simulink model "test_mdl_NI"  (R2018a)
settings: Solver=VariableStepAuto  StartTime=0.0  StopTime=10.0  RelTol=1e-3
(part 22 of 24)

== system test_mdl_NI/CAN_Signal/GWM/Other_GWMTx/APIM_Request_Signals_FD1/CbnCmrtPrefListIndx_Rq ==
  in : Inport
  out : Outport
  wires:
  in/1 -> out/1

== system test_mdl_NI/CAN_Signal/GWM/Other_GWMTx/APIM_Request_Signals_FD1/CbnCmrtPrefLstNmItm_Rq ==
  in : Inport
  out : Outport
  wires:
  in/1 -> out/1

== system test_mdl_NI/CAN_Signal/GWM/Other_GWMTx/APIM_Request_Signals_FD1/ChargePortPwr_Rq ==
  in : Inport
  out : Outport
  wires:
  in/1 -> out/1

== system test_mdl_NI/CAN_Signal/GWM/Other_GWMTx/APIM_Request_Signals_FD1/ChrgStatDsply_D_Rq ==
  in : Inport
  out : Outport
  wires:
  in/1 -> out/1

== system test_mdl_NI/CAN_Signal/GWM/Other_GWMTx/APIM_Request_Signals_FD1/FactoryReset_Rq ==
  in : Inport
  out : Outport
  wires:
  in/1 -> out/1

== system test_mdl_NI/CAN_Signal/GWM/Other_GWMTx/APIM_Request_Signals_FD1/LongTermParking_Rq ==
  in : Inport
  out : Outport
  wires:
  in/1 -> out/1

== system test_mdl_NI/CAN_Signal/GWM/Other_GWMTx/APIM_Request_Signals_FD1/ModemReset_D_Rq ==
  in : Inport
  out : Outport
  wires:
  in/1 -> out/1

== system test_mdl_NI/CAN_Signal/GWM/Other_GWMTx/APIM_Request_Signals_FD1/NextUsageTimeToggle_Rq ==
  in : Inport
  out : Outport
  wires:
  in/1 -> out/1

== system test_mdl_NI/CAN_Signal/GWM/Other_GWMTx/APIM_Request_Signals_FD1/OffPeakTimeSetHR_Rq ==
  in : Inport
  out : Outport
  wires:
  in/1 -> out/1

== system test_mdl_NI/CAN_Signal/GWM/Other_GWMTx/APIM_Request_Signals_FD1/OffPeakTimeSetMin_Rq ==
  in : Inport
  out : Outport
  wires:
  in/1 -> out/1

== system test_mdl_NI/CAN_Signal/GWM/Other_GWMTx/APIM_Request_Signals_FD1/StopStrtDrvMde_B_RqBtn3 ==
  in : Inport
  out : Outport
  wires:
  in/1 -> out/1

== system test_mdl_NI/CAN_Signal/GWM/Other_GWMTx/APIM_Request_Signals_FD1/TCU_ESN_D_Rq ==
  in : Inport
  out : Outport
  wires:
  in/1 -> out/1

== system test_mdl_NI/CAN_Signal/GWM/Other_GWMTx/APIM_Send_Signals1_FD1/APIM_ActiveTrackNum_St ==
  in : Inport
  out : Outport
  wires:
  in/1 -> out/1

== system test_mdl_NI/CAN_Signal/GWM/Other_GWMTx/APIM_Send_Signals1_FD1/APIM_NumberofTracks_St ==
  in : Inport
  out : Outport
  wires:
  in/1 -> out/1

== system test_mdl_NI/CAN_Signal/GWM/Other_GWMTx/APIM_Send_Signals1_FD1/AutoHoldSwtch_D_Stat3 ==
  in : Inport
  out : Outport
  wires:
  in/1 -> out/1

== system test_mdl_NI/CAN_Signal/GWM/Other_GWMTx/APIM_Send_Signals1_FD1/CenterStackRing_D_Actl ==
  in : Inport
  out : Outport
  wires:
  in/1 -> out/1

== system test_mdl_NI/CAN_Signal/GWM/Other_GWMTx/APIM_Send_Signals1_FD1/ChrgCordUnlock_B_Rq ==
  in : Inport
  out : Outport
  wires:
  in/1 -> out/1

== system test_mdl_NI/CAN_Signal/GWM/Other_GWMTx/APIM_Send_Signals1_FD1/TrlrAidCancl_B_Rq ==
  in : Inport
  out : Outport
  wires:
  in/1 -> out/1

== system test_mdl_NI/CAN_Signal/GWM/Other_GWMTx/APIM_Send_Signals1_FD1/TrlrAidSetup_D_Stat ==
  in : Inport
  out : Outport
  wires:
  in/1 -> out/1

== system test_mdl_NI/CAN_Signal/GWM/Other_GWMTx/APIM_Send_Signals1_FD1/TrlrTrgtAcquire_D_Rq ==
  in : Inport
  out : Outport
  wires:
  in/1 -> out/1

== system test_mdl_NI/CAN_Signal/GWM/Other_GWMTx/APIM_Send_Signals1_FD1/ValetMode_D_Stat ==
  in : Inport
  out : Outport
  wires:
  in/1 -> out/1

== system test_mdl_NI/CAN_Signal/GWM/Other_GWMTx/APIM_Send_Signals_2_FD1/OnbChrgClearAll_B_Rq ==
  in : Inport
  out : Outport
  wires:
  in/1 -> out/1

== system test_mdl_NI/CAN_Signal/GWM/Other_GWMTx/APIM_Send_Signals_2_FD1/OnbChrgGoTDelete_B_Rq ==
  in : Inport
  out : Outport
  wires:
  in/1 -> out/1

== system test_mdl_NI/CAN_Signal/GWM/Other_GWMTx/APIM_Send_Signals_2_FD1/OnbChrgGoTElement_D_Rq ==
  in : Inport
  out : Outport
  wires:
  in/1 -> out/1

== system test_mdl_NI/CAN_Signal/GWM/Other_GWMTx/APIM_Send_Signals_2_FD1/OnbChrgGoTExtHtr_D_Rq ==
  in : Inport
  out : Outport
  wires:
  in/1 -> out/1

== system test_mdl_NI/CAN_Signal/GWM/Other_GWMTx/APIM_Send_Signals_2_FD1/OnbChrgGoTHr_T_Rq ==
  in : Inport
  out : Outport
  wires:
  in/1 -> out/1

== system test_mdl_NI/CAN_Signal/GWM/Other_GWMTx/APIM_Send_Signals_2_FD1/OnbChrgGoTMnte_D_Rq ==
  in : Inport
  out : Outport
  wires:
  in/1 -> out/1

== system test_mdl_NI/CAN_Signal/GWM/Other_GWMTx/APIM_Send_Signals_2_FD1/OnbChrgGoTOn_D_Rq ==
  in : Inport
  out : Outport
  wires:
  in/1 -> out/1

== system test_mdl_NI/CAN_Signal/GWM/Other_GWMTx/APIM_Send_Signals_2_FD1/OnbChrgGoTPrcond_D_Rq ==
  in : Inport
  out : Outport
  wires:
  in/1 -> out/1

== system test_mdl_NI/CAN_Signal/GWM/Other_GWMTx/APIM_Send_Signals_2_FD1/OnbChrgGoTTouch_D_Rq ==
  in : Inport
  out : Outport
  wires:
  in/1 -> out/1

== system test_mdl_NI/CAN_Signal/GWM/Other_GWMTx/APIM_Send_Signals_2_FD1/OnbChrgGoTUpdate_B_Rq ==
  in : Inport
  out : Outport
  wires:
  in/1 -> out/1

== system test_mdl_NI/CAN_Signal/GWM/Other_GWMTx/APIM_Send_Signals_2_FD1/OtaTrg_D_Stat ==
  in : Inport
  out : Outport
  wires:
  in/1 -> out/1

== system test_mdl_NI/CAN_Signal/GWM/Other_GWMTx/APIM_Send_Signals_2_FD1/PaakMyKey_D_Rq ==
  in : Inport
  out : Outport
  wires:
  in/1 -> out/1

== system test_mdl_NI/CAN_Signal/GWM/Other_GWMTx/APIM_Send_Signals_2_FD1/TCU_Final_Actvtn_St ==
  in : Inport
  out : Outport
  wires:
  in/1 -> out/1

== system test_mdl_NI/CAN_Signal/GWM/Other_GWMTx/APIM_Send_Signals_2_FD1/TCU_Init_Actvtn_St ==
  in : Inport
  out : Outport
  wires:
  in/1 -> out/1

== system test_mdl_NI/CAN_Signal/GWM/Other_GWMTx/APIM_Send_Signals_2_FD1/TrlrAidMde_D_Rq ==
  in : Inport
  out : Outport
  wires:
  in/1 -> out/1

== system test_mdl_NI/CAN_Signal/GWM/Other_GWMTx/ActiveFrontStrg_Stat2_FD1/SteWhlRelCalib_An_Sns ==
  in : Inport
  out : Outport
  wires:
  in/1 -> out/1

== system test_mdl_NI/CAN_Signal/GWM/Other_GWMTx/ActiveFrontStrg_Stat2_FD1/SteWhlRelCalib_T_Actl ==
  in : Inport
  out : Outport
  wires:
  in/1 -> out/1

== system test_mdl_NI/CAN_Signal/GWM/Other_GWMTx/ActiveFrontStrg_Stat_FD1/SteWhlBrkAnActl_No_Cnt ==
  in : Inport
  out : Outport
  wires:
  in/1 -> out/1

== system test_mdl_NI/CAN_Signal/GWM/Other_GWMTx/ActiveFrontStrg_Stat_FD1/SteWhlBrkAnActl_No_Cs ==
  in : Inport
  out : Outport
  wires:
  in/1 -> out/1

== system test_mdl_NI/CAN_Signal/GWM/Other_GWMTx/ActiveFrontStrg_Stat_FD1/SteWhlBrkOffst_An_Actl ==
  in : Inport
  out : Outport
  wires:
  in/1 -> out/1

== system test_mdl_NI/CAN_Signal/GWM/Other_GWMTx/ActiveFrontStrg_Stat_FD1/SteWhlOffstRq_D_Stat ==
  in : Inport
  out : Outport
  wires:
  in/1 -> out/1

== system test_mdl_NI/CAN_Signal/GWM/Other_GWMTx/ActiveFrontStrg_Stat_FD1/SteWhlOffst_An_TotActl ==
  in : Inport
  out : Outport
  wires:
  in/1 -> out/1

== system test_mdl_NI/CAN_Signal/GWM/Other_GWMTx/AllTerrainControlData_FD1/SelDrvMdeCnt_D_Stat ==
  in : Inport
  out : Outport
  wires:
  in/1 -> out/1

== system test_mdl_NI/CAN_Signal/GWM/Other_GWMTx/AllTerrainControlData_FD1/SelDrvMdeSwtchOk_D_Stat ==
  in : Inport
  out : Outport
  wires:
  in/1 -> out/1

== system test_mdl_NI/CAN_Signal/GWM/Other_GWMTx/AllTerrainControlData_FD1/SelDrvMdeSwtch_D_Stat ==
  in : Inport
  out : Outport
  wires:
  in/1 -> out/1

== system test_mdl_NI/CAN_Signal/GWM/Other_GWMTx/AllTerrainControlData_FD1/SelDrvMdeSwtch_No_Actl ==
  in : Inport
  out : Outport
  wires:
  in/1 -> out/1

== system test_mdl_NI/CAN_Signal/GWM/Other_GWMTx/All_Terrain_Data_FD1/TerrMde_D_RqDrv ==
  in : Inport
  out : Outport
  wires:
  in/1 -> out/1

== system test_mdl_NI/CAN_Signal/GWM/Other_GWMTx/All_Terrain_Data_FD1/TerrStat_D_RqDsply ==
  in : Inport
  out : Outport
  wires:
  in/1 -> out/1

== system test_mdl_NI/CAN_Signal/GWM/Other_GWMTx/BCM_Lamp_Stat_FD1/BrkWarnInd_B_Rq ==
  in : Inport
  out : Outport
  wires:
  in/1 -> out/1

== system test_mdl_NI/CAN_Signal/GWM/Other_GWMTx/BCM_Lamp_Stat_FD1/Brk_Fluid_Lvl_Low ==
  in : Inport
  out : Outport
  wires:
  in/1 -> out/1

== system test_mdl_NI/CAN_Signal/GWM/Other_GWMTx/BCM_Lamp_Stat_FD1/Courtesy_BSave_Stat ==
  in : Inport
  out : Outport
  wires:
  in/1 -> out/1

== system test_mdl_NI/CAN_Signal/GWM/Other_GWMTx/BCM_Lamp_Stat_FD1/Courtesy_Delay_Status ==
  in : Inport
  out : Outport
  wires:
  in/1 -> out/1

== system test_mdl_NI/CAN_Signal/GWM/Other_GWMTx/BCM_Lamp_Stat_FD1/CrnrLghtLeft_Pc_Rq ==
  in : Inport
  out : Outport
  wires:
  in/1 -> out/1

== system test_mdl_NI/CAN_Signal/GWM/Other_GWMTx/BCM_Lamp_Stat_FD1/CrnrLghtRight_Pc_Rq ==
  in : Inport
  out : Outport
  wires:
  in/1 -> out/1

== system test_mdl_NI/CAN_Signal/GWM/Other_GWMTx/BCM_Lamp_Stat_FD1/DayRnngLampOn_B_Stat ==
  in : Inport
  out : Outport
  wires:
  in/1 -> out/1

== system test_mdl_NI/CAN_Signal/GWM/Other_GWMTx/BCM_Lamp_Stat_FD1/DrTgateLck_D_Stat ==
  in : Inport
  out : Outport
  wires:
  in/1 -> out/1

== system test_mdl_NI/CAN_Signal/GWM/Other_GWMTx/BCM_Lamp_Stat_FD1/Dr_Courtesy_Light_Stat ==
  in : Inport
  out : Outport
  wires:
  in/1 -> out/1

== system test_mdl_NI/CAN_Signal/GWM/Other_GWMTx/BCM_Lamp_Stat_FD1/HeadLampLoActv_B_Stat ==
  in : Inport
  out : Outport
  wires:
  in/1 -> out/1

== system test_mdl_NI/CAN_Signal/GWM/Other_GWMTx/BCM_Lamp_Stat_FD1/HeadLampLoFlOn_B_Stat ==
  in : Inport
  out : Outport
  wires:
  in/1 -> out/1

== system test_mdl_NI/CAN_Signal/GWM/Other_GWMTx/BCM_Lamp_Stat_FD1/HeadLampLoFrOn_B_Stat ==
  in : Inport
  out : Outport
  wires:
  in/1 -> out/1

== system test_mdl_NI/CAN_Signal/GWM/Other_GWMTx/BCM_Lamp_Stat_FD1/HeadLampLoOut_B_Stat ==
  in : Inport
  out : Outport
  wires:
  in/1 -> out/1

== system test_mdl_NI/CAN_Signal/GWM/Other_GWMTx/BCM_Lamp_Stat_FD1/HeadLghtHiFdbck_D_Stat ==
  in : Inport
  out : Outport
  wires:
  in/1 -> out/1

== system test_mdl_NI/CAN_Signal/GWM/Other_GWMTx/BCM_Lamp_Stat_FD1/HeadLghtHiOn_B_Stat ==
  in : Inport
  out : Outport
  wires:
  in/1 -> out/1

== system test_mdl_NI/CAN_Signal/GWM/Other_GWMTx/BCM_Lamp_Stat_FD1/HeadLghtSwtch_D_Stat ==
  in : Inport
  out : Outport
  wires:
  in/1 -> out/1

== system test_mdl_NI/CAN_Signal/GWM/Other_GWMTx/BCM_Lamp_Stat_FD1/Headlamp_On_Wrning_Cmd ==
  in : Inport
  out : Outport
  wires:
  in/1 -> out/1

== system test_mdl_NI/CAN_Signal/GWM/Other_GWMTx/BCM_Lamp_Stat_FD1/HomeSafeLtChime_B_Rq ==
  in : Inport
  out : Outport
  wires:
  in/1 -> out/1

== system test_mdl_NI/CAN_Signal/GWM/Other_GWMTx/BCM_Lamp_Stat_FD1/Illuminated_Entry_Stat ==
  in : Inport
  out : Outport
  wires:
  in/1 -> out/1

== system test_mdl_NI/CAN_Signal/GWM/Other_GWMTx/BCM_Lamp_Stat_FD1/ImpactEvntFdbck_D_Stat ==
  in : Inport
  out : Outport
  wires:
  in/1 -> out/1

== system test_mdl_NI/CAN_Signal/GWM/Other_GWMTx/BCM_Lamp_Stat_FD1/KeyInIgnWarn_B_Cmd ==
  in : Inport
  out : Outport
  wires:
  in/1 -> out/1

== system test_mdl_NI/CAN_Signal/GWM/Other_GWMTx/BCM_Lamp_Stat_FD1/Park_Brake_Chime_Rqst ==
  in : Inport
  out : Outport
  wires:
  in/1 -> out/1

== system test_mdl_NI/CAN_Signal/GWM/Other_GWMTx/BCM_Lamp_Stat_FD1/PerimeterAlarmChimeRq ==
  in : Inport
  out : Outport
  wires:
  in/1 -> out/1

== system test_mdl_NI/CAN_Signal/GWM/Other_GWMTx/BCM_Lamp_Stat_FD1/Perimeter_Alarm_Status ==
  in : Inport
  out : Outport
  wires:
  in/1 -> out/1

== system test_mdl_NI/CAN_Signal/GWM/Other_GWMTx/BCM_Lamp_Stat_FD1/PrkLght_D_Stat ==
  in : Inport
  out : Outport
  wires:
  in/1 -> out/1

== system test_mdl_NI/CAN_Signal/GWM/Other_GWMTx/BCM_Lamp_Stat_FD1/PrkLightChime_B_Rq ==
  in : Inport
  out : Outport
  wires:
  in/1 -> out/1

== system test_mdl_NI/CAN_Signal/GWM/Other_GWMTx/BCM_Lamp_Stat_FD1/PudLampDrv_D_Rq ==
  in : Inport
  out : Outport
  wires:
  in/1 -> out/1

== system test_mdl_NI/CAN_Signal/GWM/Other_GWMTx/BCM_Lamp_Stat_FD1/PudLampPsngr_D_Rq ==
  in : Inport
  out : Outport
  wires:
  in/1 -> out/1

== system test_mdl_NI/CAN_Signal/GWM/Other_GWMTx/BCM_Lamp_Stat_FD1/PudLamp_D_Rq ==
  in : Inport
  out : Outport
  wires:
  in/1 -> out/1

== system test_mdl_NI/CAN_Signal/GWM/Other_GWMTx/BCM_Lamp_Stat_FD1/ReducedGuard_D_Stat ==
  in : Inport
  out : Outport
  wires:
  in/1 -> out/1

== system test_mdl_NI/CAN_Signal/GWM/Other_GWMTx/BCM_Lamp_Stat_FD1/RvrseLghtOn_B_Stat ==
  in : Inport
  out : Outport
  wires:
  in/1 -> out/1

== system test_mdl_NI/CAN_Signal/GWM/Other_GWMTx/BCM_Lamp_Stat_FD1/StopLghtOn_B_Stat ==
  in : Inport
  out : Outport
  wires:
  in/1 -> out/1

== system test_mdl_NI/CAN_Signal/GWM/Other_GWMTx/BCM_Lamp_Stat_FD1/TrnNotInPrkChime_B_Rq ==
  in : Inport
  out : Outport
  wires:
  in/1 -> out/1

== system test_mdl_NI/CAN_Signal/GWM/Other_GWMTx/BCM_Lamp_Stat_FD1/WndwGlbl_D_Cmd ==
  in : Inport
  out : Outport
  wires:
  in/1 -> out/1

== system test_mdl_NI/CAN_Signal/GWM/Other_GWMTx/BCM_Lamp_Stat_FD1/WrlssAcsyChrgInhbt_B_Rq ==
  in : Inport
  out : Outport
  wires:
  in/1 -> out/1

== system test_mdl_NI/CAN_Signal/GWM/Other_GWMTx/BatteryCharge_Data2_FD1/ChrgCrdLck_D_Falt ==
  in : Inport
  out : Outport
  wires:
  in/1 -> out/1

== system test_mdl_NI/CAN_Signal/GWM/Other_GWMTx/Battery_Mgmt_24V_FD1/BattULo24Soc_Pc_Actl ==
  in : Inport
  out : Outport
  wires:
  in/1 -> out/1

== system test_mdl_NI/CAN_Signal/GWM/Other_GWMTx/Battery_Mgmt_24V_FD1/BattULo24State_D_Qlty ==
  in : Inport
  out : Outport
  wires:
  in/1 -> out/1

== system test_mdl_NI/CAN_Signal/GWM/Other_GWMTx/Battery_Mgmt_24V_FD1/BattULo24_Ah_DeltaRide ==
  in : Inport
  out : Outport
  wires:
  in/1 -> out/1

== system test_mdl_NI/CAN_Signal/GWM/Other_GWMTx/Battery_Mgmt_24V_FD1/BattULo24_B_Falt ==
  in : Inport
  out : Outport
  wires:
  in/1 -> out/1

== system test_mdl_NI/CAN_Signal/GWM/Other_GWMTx/Battery_Mgmt_24V_FD1/BattULo24_I_Actl ==
  in : Inport
  out : Outport
  wires:
  in/1 -> out/1

== system test_mdl_NI/CAN_Signal/GWM/Other_GWMTx/Battery_Mgmt_2_FD1/BattULoChrg_D_Rq ==
  in : Inport
  out : Outport
  wires:
  in/1 -> out/1

== system test_mdl_NI/CAN_Signal/GWM/Other_GWMTx/Battery_Mgmt_2_FD1/BattULoSrvc_T_Actl ==
  in : Inport
  out : Outport
  wires:
  in/1 -> out/1

== system test_mdl_NI/CAN_Signal/GWM/Other_GWMTx/Battery_Mgmt_2_FD1/Batt_Crit_SoC_B ==
  in : Inport
  out : Outport
  wires:
  in/1 -> out/1

== system test_mdl_NI/CAN_Signal/GWM/Other_GWMTx/Battery_Mgmt_2_FD1/Batt_Lo_SoC_B ==
  in : Inport
  out : Outport
  wires:
  in/1 -> out/1

== system test_mdl_NI/CAN_Signal/GWM/Other_GWMTx/Battery_Mgmt_2_FD1/ChargeMode ==
  in : Inport
  out : Outport
  wires:
  in/1 -> out/1

== system test_mdl_NI/CAN_Signal/GWM/Other_GWMTx/Battery_Mgmt_2_FD1/EngStrtInhbt_B_RqBatt ==
  in : Inport
  out : Outport
  wires:
  in/1 -> out/1

== system test_mdl_NI/CAN_Signal/GWM/Other_GWMTx/Battery_Mgmt_2_FD1/IdleSpeedIncrease_El ==
  in : Inport
  out : Outport
  wires:
  in/1 -> out/1

== system test_mdl_NI/CAN_Signal/GWM/Other_GWMTx/Battery_Mgmt_2_FD1/PeriodicElLoad_B_Stat ==
  in : Inport
  out : Outport
  wires:
  in/1 -> out/1

== system test_mdl_NI/CAN_Signal/GWM/Other_GWMTx/Battery_Mgmt_2_FD1/PwSysULoFalt_D_Stat ==
  in : Inport
  out : Outport
  wires:
  in/1 -> out/1

== system test_mdl_NI/CAN_Signal/GWM/Other_GWMTx/Battery_Mgmt_2_FD1/Shed_Drain_Eng_Off_B ==
  in : Inport
  out : Outport
  wires:
  in/1 -> out/1

== system test_mdl_NI/CAN_Signal/GWM/Other_GWMTx/Battery_Mgmt_2_FD1/Shed_Feature_Group_ID ==
  in : Inport
  out : Outport
  wires:
  in/1 -> out/1

== system test_mdl_NI/CAN_Signal/GWM/Other_GWMTx/Battery_Mgmt_2_FD1/Shed_Level_Req ==
  in : Inport
  out : Outport
  wires:
  in/1 -> out/1

== system test_mdl_NI/CAN_Signal/GWM/Other_GWMTx/Battery_Mgmt_2_FD1/Shed_T_Eng_Off_B ==
  in : Inport
  out : Outport
  wires:
  in/1 -> out/1

== system test_mdl_NI/CAN_Signal/GWM/Other_GWMTx/Battery_Mgmt_2_FD1/ULoRgenTestMde_B_Rq ==
  in : Inport
  out : Outport
  wires:
  in/1 -> out/1

== system test_mdl_NI/CAN_Signal/GWM/Other_GWMTx/Battery_Mgmt_3_FD1/BSBattQCapAh ==
  in : Inport
  out : Outport
  wires:
  in/1 -> out/1

== system test_mdl_NI/CAN_Signal/GWM/Other_GWMTx/Battery_Mgmt_3_FD1/BSBattQDeltaRideAh ==
  in : Inport
  out : Outport
  wires:
  in/1 -> out/1

== system test_mdl_NI/CAN_Signal/GWM/Other_GWMTx/Battery_Mgmt_3_FD1/BSBattSOC ==
  in : Inport
  out : Outport
  wires:
  in/1 -> out/1

== system test_mdl_NI/CAN_Signal/GWM/Other_GWMTx/Battery_Mgmt_3_FD1/BSFault ==
  in : Inport
  out : Outport
  wires:
  in/1 -> out/1

== system test_mdl_NI/CAN_Signal/GWM/Other_GWMTx/Battery_Mgmt_3_FD1/BattULo2_Te_Actl ==
  in : Inport
  out : Outport
  wires:
  in/1 -> out/1

== system test_mdl_NI/CAN_Signal/GWM/Other_GWMTx/Battery_Mgmt_3_FD1/BattULoChrg_URate_RqMx ==
  in : Inport
  out : Outport
  wires:
  in/1 -> out/1

== system test_mdl_NI/CAN_Signal/GWM/Other_GWMTx/Battery_Mgmt_3_FD1/BattULoChrg_U_RqMn ==
  in : Inport
  out : Outport
  wires:
  in/1 -> out/1

== system test_mdl_NI/CAN_Signal/GWM/Other_GWMTx/Battery_Mgmt_3_FD1/BattULoChrg_U_RqMx ==
  in : Inport
  out : Outport
  wires:
  in/1 -> out/1

== system test_mdl_NI/CAN_Signal/GWM/Other_GWMTx/Battery_Mgmt_3_FD1/BattULoState_D_Qlty ==
  in : Inport
  out : Outport
  wires:
  in/1 -> out/1

== system test_mdl_NI/CAN_Signal/GWM/Other_GWMTx/Battery_Mgmt_4_FD1/BattULoAuxSoc_Pc_Actl ==
  in : Inport
  out : Outport
  wires:
  in/1 -> out/1

== system test_mdl_NI/CAN_Signal/GWM/Other_GWMTx/Battery_Mgmt_4_FD1/BattULoAux_B_Falt ==
  in : Inport
  out : Outport
  wires:
  in/1 -> out/1

== system test_mdl_NI/CAN_Signal/GWM/Other_GWMTx/Battery_Mgmt_4_FD1/BattULoAux_D_Qlty ==
  in : Inport
  out : Outport
  wires:
  in/1 -> out/1

== system test_mdl_NI/CAN_Signal/GWM/Other_GWMTx/Battery_Mgmt_4_FD1/BattULoAux_I_Actl ==
  in : Inport
  out : Outport
  wires:
  in/1 -> out/1

== system test_mdl_NI/CAN_Signal/GWM/Other_GWMTx/Battery_Mgmt_4_FD1/BattULoAux_U_Actl ==
  in : Inport
  out : Outport
  wires:
  in/1 -> out/1

== system test_mdl_NI/CAN_Signal/GWM/Other_GWMTx/Battery_Mgmt_4_FD1/BattULoCrnkBelt_U_Pred ==
  in : Inport
  out : Outport
  wires:
  in/1 -> out/1

== system test_mdl_NI/CAN_Signal/GWM/Other_GWMTx/Battery_Mgmt_4_FD1/BattULoCrnkStrt_U_Pred ==
  in : Inport
  out : Outport
  wires:
  in/1 -> out/1

== system test_mdl_NI/CAN_Signal/GWM/Other_GWMTx/Battery_Traction_1_FD1/BattTracMil_D_Rq ==
  in : Inport
  out : Outport
  wires:
  in/1 -> out/1

== system test_mdl_NI/CAN_Signal/GWM/Other_GWMTx/Battery_Traction_1_FD1/BattTracOffFst_D_Actl ==
  in : Inport
  out : Outport
  wires:
  in/1 -> out/1

== system test_mdl_NI/CAN_Signal/GWM/Other_GWMTx/Battery_Traction_1_FD1/BattTracOff_B_Actl ==
  in : Inport
  out : Outport
  wires:
  in/1 -> out/1

== system test_mdl_NI/CAN_Signal/GWM/Other_GWMTx/Battery_Traction_1_FD1/BattTrac_I_Actl ==
  in : Inport
  out : Outport
  wires:
  in/1 -> out/1

== system test_mdl_NI/CAN_Signal/GWM/Other_GWMTx/Battery_Traction_1_FD1/BattTrac_U_Actl ==
  in : Inport
  out : Outport
  wires:
  in/1 -> out/1

== system test_mdl_NI/CAN_Signal/GWM/Other_GWMTx/Battery_Traction_1_FD1/BattTrac_U_LimHi ==
  in : Inport
  out : Outport
  wires:
  in/1 -> out/1

== system test_mdl_NI/CAN_Signal/GWM/Other_GWMTx/Battery_Traction_1_FD1/BattTrac_U_LimLo ==
  in : Inport
  out : Outport
  wires:
  in/1 -> out/1

== system test_mdl_NI/CAN_Signal/GWM/Other_GWMTx/Battery_Traction_1_FD1/VehStrtInhbt_B_RqBatt ==
  in : Inport
  out : Outport
  wires:
  in/1 -> out/1

== system test_mdl_NI/CAN_Signal/GWM/Other_GWMTx/Battery_Traction_3_FD1/BattTracClnt_Te_Actl ==
  in : Inport
  out : Outport
  wires:
  in/1 -> out/1

== system test_mdl_NI/CAN_Signal/GWM/Other_GWMTx/Battery_Traction_3_FD1/BattTracSoc_Pc_LimHi ==
  in : Inport
  out : Outport
  wires:
  in/1 -> out/1

== system test_mdl_NI/CAN_Signal/GWM/Other_GWMTx/Battery_Traction_3_FD1/BattTracSoc_Pc_LimLo ==
  in : Inport
  out : Outport
  wires:
  in/1 -> out/1

== system test_mdl_NI/CAN_Signal/GWM/Other_GWMTx/Battery_Traction_3_FD1/BattTracSoc_Pc_MnPrtct ==
  in : Inport
  out : Outport
  wires:
  in/1 -> out/1

== system test_mdl_NI/CAN_Signal/GWM/Other_GWMTx/Battery_Traction_3_FD1/BattTracSoc_Pc_MxPrtct ==
  in : Inport
  out : Outport
  wires:
  in/1 -> out/1

== system test_mdl_NI/CAN_Signal/GWM/Other_GWMTx/Battery_Traction_3_FD1/BattTracSrvcRqd_B_Rq ==
  in : Inport
  out : Outport
  wires:
  in/1 -> out/1

== system test_mdl_NI/CAN_Signal/GWM/Other_GWMTx/Battery_Traction_3_FD1/BattTracWarnLamp_B_Rq ==
  in : Inport
  out : Outport
  wires:
  in/1 -> out/1

== system test_mdl_NI/CAN_Signal/GWM/Other_GWMTx/Battery_Traction_4_FD1/BattTracDiagClr_B_Rq ==
  in : Inport
  out : Outport
  wires:
  in/1 -> out/1

== system test_mdl_NI/CAN_Signal/GWM/Other_GWMTx/Battery_Traction_4_FD1/BattTracSoc2_Pc_Actl ==
  in : Inport
  out : Outport
  wires:
  in/1 -> out/1

== system test_mdl_NI/CAN_Signal/GWM/Other_GWMTx/Battery_Traction_4_FD1/BattTrac_Te_Actl ==
  in : Inport
  out : Outport
  wires:
  in/1 -> out/1

== system test_mdl_NI/CAN_Signal/GWM/Other_GWMTx/Battery_Traction_5_FD1/BattTrac2_Pw_ChrgInst ==
  in : Inport
  out : Outport
  wires:
  in/1 -> out/1

== system test_mdl_NI/CAN_Signal/GWM/Other_GWMTx/Battery_Traction_5_FD1/BattTrac2_Pw_DchrgInst ==
  in : Inport
  out : Outport
  wires:
  in/1 -> out/1

== system test_mdl_NI/CAN_Signal/GWM/Other_GWMTx/Battery_Traction_5_FD1/BattTrac2_Pw_LimChrg ==
  in : Inport
  out : Outport
  wires:
  in/1 -> out/1

== system test_mdl_NI/CAN_Signal/GWM/Other_GWMTx/Battery_Traction_5_FD1/BattTrac2_Pw_LimDchrg ==
  in : Inport
  out : Outport
  wires:
  in/1 -> out/1

== system test_mdl_NI/CAN_Signal/GWM/Other_GWMTx/Battery_Traction_6_FD1/BattTracClntPmp_D_Stat ==
  in : Inport
  out : Outport
  wires:
  in/1 -> out/1

== system test_mdl_NI/CAN_Signal/GWM/Other_GWMTx/Battery_Traction_6_FD1/BattTracCnnct_D_Cmd ==
  in : Inport
  out : Outport
  wires:
  in/1 -> out/1

== system test_mdl_NI/CAN_Signal/GWM/Other_GWMTx/Battery_Traction_6_FD1/BattTracDcdcDis_B_Rq ==
  in : Inport
  out : Outport
  wires:
  in/1 -> out/1

== system test_mdl_NI/CAN_Signal/GWM/Other_GWMTx/Battery_Traction_6_FD1/BattTracDelta_Te_Actl ==
  in : Inport
  out : Outport
  wires:
  in/1 -> out/1

== system test_mdl_NI/CAN_Signal/GWM/Other_GWMTx/Battery_Traction_6_FD1/BattTracHvilOpen_B_Stat ==
  in : Inport
  out : Outport
  wires:
  in/1 -> out/1

== system test_mdl_NI/CAN_Signal/GWM/Other_GWMTx/Battery_Traction_6_FD1/HtrnClntPump_D_Stat ==
  in : Inport
  out : Outport
  wires:
  in/1 -> out/1

== system test_mdl_NI/CAN_Signal/GWM/Other_GWMTx/BodyInfo_3_FD1/Backlit_LED_Status ==
  in : Inport
  out : Outport
  wires:
  in/1 -> out/1

== system test_mdl_NI/CAN_Signal/GWM/Other_GWMTx/BodyInfo_3_FD1/BodySrvcRqd_B_Rq ==
  in : Inport
  out : Outport
  wires:
  in/1 -> out/1

== system test_mdl_NI/CAN_Signal/GWM/Other_GWMTx/BodyInfo_3_FD1/CrashEvnt_D_Stat ==
  in : Inport
  out : Outport
  wires:
  in/1 -> out/1

== system test_mdl_NI/CAN_Signal/GWM/Other_GWMTx/BodyInfo_3_FD1/Day_Night_Status ==
  in : Inport
  out : Outport
  wires:
  in/1 -> out/1

== system test_mdl_NI/CAN_Signal/GWM/Other_GWMTx/BodyInfo_3_FD1/Delay_Accy ==
  in : Inport
  out : Outport
  wires:
  in/1 -> out/1

== system test_mdl_NI/CAN_Signal/GWM/Other_GWMTx/BodyInfo_3_FD1/DimmingLvlEvnt_No_Actl ==
  in : Inport
  out : Outport
  wires:
  in/1 -> out/1

== system test_mdl_NI/CAN_Signal/GWM/Other_GWMTx/BodyInfo_3_FD1/Dimming_Lvl ==
  in : Inport
  out : Outport
  wires:
  in/1 -> out/1

== system test_mdl_NI/CAN_Signal/GWM/Other_GWMTx/BodyInfo_3_FD1/DrStatDrvErrCnt_B_Stat ==
  in : Inport
  out : Outport
  wires:
  in/1 -> out/1

== system test_mdl_NI/CAN_Signal/GWM/Other_GWMTx/BodyInfo_3_FD1/DrStatDrv_B_Actl ==
  in : Inport
  out : Outport
  wires:
  in/1 -> out/1

== system test_mdl_NI/CAN_Signal/GWM/Other_GWMTx/BodyInfo_3_FD1/DrStatHood_B_Actl ==
  in : Inport
  out : Outport
  wires:
  in/1 -> out/1

== system test_mdl_NI/CAN_Signal/GWM/Other_GWMTx/BodyInfo_3_FD1/DrStatInnrTgate_B_Actl ==
  in : Inport
  out : Outport
  wires:
  in/1 -> out/1

== system test_mdl_NI/CAN_Signal/GWM/Other_GWMTx/BodyInfo_3_FD1/DrStatPsngr_B_Actl ==
  in : Inport
  out : Outport
  wires:
  in/1 -> out/1

== system test_mdl_NI/CAN_Signal/GWM/Other_GWMTx/BodyInfo_3_FD1/DrStatRl_B_Actl ==
  in : Inport
  out : Outport
  wires:
  in/1 -> out/1

== system test_mdl_NI/CAN_Signal/GWM/Other_GWMTx/BodyInfo_3_FD1/DrStatRr_B_Actl ==
  in : Inport
  out : Outport
  wires:
  in/1 -> out/1

== system test_mdl_NI/CAN_Signal/GWM/Other_GWMTx/BodyInfo_3_FD1/DrStatTgate_B_Actl ==
  in : Inport
  out : Outport
  wires:
  in/1 -> out/1

== system test_mdl_NI/CAN_Signal/GWM/Other_GWMTx/BodyInfo_3_FD1/FogLghtFrontOn_B_Stat ==
  in : Inport
  out : Outport
  wires:
  in/1 -> out/1

== system test_mdl_NI/CAN_Signal/GWM/Other_GWMTx/BodyInfo_3_FD1/FogLghtRearOn_B_Stat ==
  in : Inport
  out : Outport
  wires:
  in/1 -> out/1

== system test_mdl_NI/CAN_Signal/GWM/Other_GWMTx/BodyInfo_3_FD1/FuelPmpInhbt_B_Stat ==
  in : Inport
  out : Outport
  wires:
  in/1 -> out/1

== system test_mdl_NI/CAN_Signal/GWM/Other_GWMTx/BodyInfo_3_FD1/IgnKeyType_D_Actl ==
  in : Inport
  out : Outport
  wires:
  in/1 -> out/1

== system test_mdl_NI/CAN_Signal/GWM/Other_GWMTx/BodyInfo_3_FD1/Ignition_Status ==
  in : Inport
  out : Outport
  wires:
  in/1 -> out/1

== system test_mdl_NI/CAN_Signal/GWM/Other_GWMTx/BodyInfo_3_FD1/Key_In_Ignition_Stat ==
  in : Inport
  out : Outport
  wires:
  in/1 -> out/1

== system test_mdl_NI/CAN_Signal/GWM/Other_GWMTx/BodyInfo_3_FD1/LifeCycMde_D_Actl ==
  in : Inport
  out : Outport
  wires:
  in/1 -> out/1

== system test_mdl_NI/CAN_Signal/GWM/Other_GWMTx/BodyInfo_3_FD1/Litval ==
  in : Inport
  out : Outport
  wires:
  in/1 -> out/1

== system test_mdl_NI/CAN_Signal/GWM/Other_GWMTx/BodyInfo_3_FD1/Parklamp_Status ==
  in : Inport
  out : Outport
  wires:
  in/1 -> out/1

== system test_mdl_NI/CAN_Signal/GWM/Other_GWMTx/BodyInfo_3_FD1/PrkBrkActv_B_Actl ==
  in : Inport
  out : Outport
  wires:
  in/1 -> out/1

== system test_mdl_NI/CAN_Signal/GWM/Other_GWMTx/BodyInfo_3_FD1/Remote_Start_Status ==
  in : Inport
  out : Outport
  wires:
  in/1 -> out/1

== system test_mdl_NI/CAN_Signal/GWM/Other_GWMTx/BodyInfo_3_FD1/TurnLghtLeftOn_B_Stat ==
  in : Inport
  out : Outport
  wires:
  in/1 -> out/1

== system test_mdl_NI/CAN_Signal/GWM/Other_GWMTx/BodyInfo_3_FD1/TurnLghtLeft_D_Rq ==
  in : Inport
  out : Outport
  wires:
  in/1 -> out/1

== system test_mdl_NI/CAN_Signal/GWM/Other_GWMTx/BodyInfo_3_FD1/TurnLghtRightOn_B_Stat ==
  in : Inport
  out : Outport
  wires:
  in/1 -> out/1

== system test_mdl_NI/CAN_Signal/GWM/Other_GWMTx/BodyInfo_3_FD1/TurnLghtRight_D_Rq ==
  in : Inport
  out : Outport
  wires:
  in/1 -> out/1

== system test_mdl_NI/CAN_Signal/GWM/Other_GWMTx/BodyInfo_3_FD1/ValetMode_D_Mem ==
  in : Inport
  out : Outport
  wires:
  in/1 -> out/1

== system test_mdl_NI/CAN_Signal/GWM/Other_GWMTx/Body_Info_10_FD1/GenericSwtch1_No_Actl ==
  in : Inport
  out : Outport
  wires:
  in/1 -> out/1

== system test_mdl_NI/CAN_Signal/GWM/Other_GWMTx/Body_Info_10_FD1/GenericSwtch2_No_Actl ==
  in : Inport
  out : Outport
  wires:
  in/1 -> out/1

== system test_mdl_NI/CAN_Signal/GWM/Other_GWMTx/Body_Info_10_FD1/GenericSwtch3_No_Actl ==
  in : Inport
  out : Outport
  wires:
  in/1 -> out/1

== system test_mdl_NI/CAN_Signal/GWM/Other_GWMTx/Body_Info_4_FD1/BattULo_I_Actl ==
  in : Inport
  out : Outport
  wires:
  in/1 -> out/1

== system test_mdl_NI/CAN_Signal/GWM/Other_GWMTx/Body_Info_4_FD1/BattULo_U_Actl ==
  in : Inport
  out : Outport
  wires:
  in/1 -> out/1

== system test_mdl_NI/CAN_Signal/GWM/Other_GWMTx/Body_Info_4_FD1/BrkTrnShifLck_B_Stat ==
  in : Inport
  out : Outport
  wires:
  in/1 -> out/1

== system test_mdl_NI/CAN_Signal/GWM/Other_GWMTx/Body_Info_4_FD1/DcacElPw_D_Rq ==
  in : Inport
  out : Outport
  wires:
  in/1 -> out/1

== system test_mdl_NI/CAN_Signal/GWM/Other_GWMTx/Body_Info_4_FD1/DriverCrankingReq ==
  in : Inport
  out : Outport
  wires:
  in/1 -> out/1

== system test_mdl_NI/CAN_Signal/GWM/Other_GWMTx/Body_Info_4_FD1/EngOff_T_Actl ==
  in : Inport
  out : Outport
  wires:
  in/1 -> out/1

== system test_mdl_NI/CAN_Signal/GWM/Other_GWMTx/Body_Info_4_FD1/FuelPumpPwr_D_Stat ==
  in : Inport
  out : Outport
  wires:
  in/1 -> out/1

== system test_mdl_NI/CAN_Signal/GWM/Other_GWMTx/Body_Info_4_FD1/PrkLckCtlAvail_T_Stat ==
  in : Inport
  out : Outport
  wires:
  in/1 -> out/1

== system test_mdl_NI/CAN_Signal/GWM/Other_GWMTx/Body_Info_4_FD1/PrkLckCtlMsgTxt_D_Rq ==
  in : Inport
  out : Outport
  wires:
  in/1 -> out/1

== system test_mdl_NI/CAN_Signal/GWM/Other_GWMTx/Body_Info_4_FD1/PrkLckCtlTow_B_Enbl ==
  in : Inport
  out : Outport
  wires:
  in/1 -> out/1

== system test_mdl_NI/CAN_Signal/GWM/Other_GWMTx/Body_Info_4_FD1/PrkLckCtlUnlck_D_Stat ==
  in : Inport
  out : Outport
  wires:
  in/1 -> out/1

== system test_mdl_NI/CAN_Signal/GWM/Other_GWMTx/Body_Info_4_FD1/PrkLckCtl_B_Enbl ==
  in : Inport
  out : Outport
  wires:
  in/1 -> out/1

== system test_mdl_NI/CAN_Signal/GWM/Other_GWMTx/Body_Info_4_FD1/PtLatchActv_B_RqBcm ==
  in : Inport
  out : Outport
  wires:
  in/1 -> out/1

== system test_mdl_NI/CAN_Signal/GWM/Other_GWMTx/Body_Info_4_FD1/ReFuelSwtchStat_D_Actl ==
  in : Inport
  out : Outport
  wires:
  in/1 -> out/1

== system test_mdl_NI/CAN_Signal/GWM/Other_GWMTx/Body_Info_4_FD1/immoSecureIdleMode ==
  in : Inport
  out : Outport
  wires:
  in/1 -> out/1

== system test_mdl_NI/CAN_Signal/GWM/Other_GWMTx/Body_Info_6_FD1/DrLatchMsgTxt_D_Rq ==
  in : Inport
  out : Outport
  wires:
  in/1 -> out/1

== system test_mdl_NI/CAN_Signal/GWM/Other_GWMTx/Body_Info_6_FD1/ElPwPoint_D_Rq ==
  in : Inport
  out : Outport
  wires:
  in/1 -> out/1

== system test_mdl_NI/CAN_Signal/GWM/Other_GWMTx/Body_Info_6_FD1/HeadLghtHiPrmsn_D_Stat ==
  in : Inport
  out : Outport
  wires:
  in/1 -> out/1

== system test_mdl_NI/CAN_Signal/GWM/Other_GWMTx/Body_Info_6_FD1/IgnPsswrdDsply_B_Rq ==
  in : Inport
  out : Outport
  wires:
  in/1 -> out/1

== system test_mdl_NI/CAN_Signal/GWM/Other_GWMTx/Body_Info_6_FD1/KeyAdmnTot_No_Cnt ==
  in : Inport
  out : Outport
  wires:
  in/1 -> out/1

== system test_mdl_NI/CAN_Signal/GWM/Other_GWMTx/Body_Info_6_FD1/KeyMykeyTot_No_Cnt ==
  in : Inport
  out : Outport
  wires:
  in/1 -> out/1

== system test_mdl_NI/CAN_Signal/GWM/Other_GWMTx/Body_Info_6_FD1/Keycode_Status ==
  in : Inport
  out : Outport
  wires:
  in/1 -> out/1

== system test_mdl_NI/CAN_Signal/GWM/Other_GWMTx/Body_Info_6_FD1/PEBackupSlot_Stats ==
  in : Inport
  out : Outport
  wires:
  in/1 -> out/1

== system test_mdl_NI/CAN_Signal/GWM/Other_GWMTx/Body_Info_6_FD1/PoliceIdlMde_D_Stat ==
  in : Inport
  out : Outport
  wires:
  in/1 -> out/1

== system test_mdl_NI/CAN_Signal/GWM/Other_GWMTx/Body_Info_6_FD1/PrmtrAlrmEvnt_D_Stat ==
  in : Inport
  out : Outport
  wires:
  in/1 -> out/1

== system test_mdl_NI/CAN_Signal/GWM/Other_GWMTx/Body_Info_6_FD1/PrsnlDevcChrgEnbl_B_Rq ==
  in : Inport
  out : Outport
  wires:
  in/1 -> out/1

== system test_mdl_NI/CAN_Signal/GWM/Other_GWMTx/Body_Info_6_FD1/SecurityMsgTxt_D_Rq ==
  in : Inport
  out : Outport
  wires:
  in/1 -> out/1

== system test_mdl_NI/CAN_Signal/GWM/Other_GWMTx/Body_Info_6_FD1/SteWhlLckMsgTxt_D_Rq ==
  in : Inport
  out : Outport
  wires:
  in/1 -> out/1

== system test_mdl_NI/CAN_Signal/GWM/Other_GWMTx/Body_Info_6_FD1/TracKeyMde_D_Stat ==
  in : Inport
  out : Outport
  wires:
  in/1 -> out/1

== system test_mdl_NI/CAN_Signal/GWM/Other_GWMTx/Body_Info_6_FD1/immoMsgTxt_D_Rq ==
  in : Inport
  out : Outport
  wires:
  in/1 -> out/1

== system test_mdl_NI/CAN_Signal/GWM/Other_GWMTx/Body_Info_8_FD1/ChrgCordLck_B_Stat ==
  in : Inport
  out : Outport
  wires:
  in/1 -> out/1

== system test_mdl_NI/CAN_Signal/GWM/Other_GWMTx/Body_Info_8_FD1/ChrgCordResp1_No_Actl ==
  in : Inport
  out : Outport
  wires:
  in/1 -> out/1

== system test_mdl_NI/CAN_Signal/GWM/Other_GWMTx/Body_Info_8_FD1/ChrgCordResp2_No_Actl ==
  in : Inport
  out : Outport
  wires:
  in/1 -> out/1

== system test_mdl_NI/CAN_Signal/GWM/Other_GWMTx/Body_Info_8_FD1/WakeAlarm0_D_Stat ==
  in : Inport
  out : Outport
  wires:
  in/1 -> out/1

== system test_mdl_NI/CAN_Signal/GWM/Other_GWMTx/Body_Info_8_FD1/WakeAlarm1_D_Stat ==
  in : Inport
  out : Outport
  wires:
  in/1 -> out/1

== system test_mdl_NI/CAN_Signal/GWM/Other_GWMTx/Body_Info_8_FD1/WakeAlarm2_D_Stat ==
  in : Inport
  out : Outport
  wires:
  in/1 -> out/1

== system test_mdl_NI/CAN_Signal/GWM/Other_GWMTx/Body_Info_8_FD1/WakeAlarm3_D_Stat ==
  in : Inport
  out : Outport
  wires:
  in/1 -> out/1

== system test_mdl_NI/CAN_Signal/GWM/Other_GWMTx/Body_Info_9_FD1/AdvStrt_D_Stat ==
  in : Inport
  out : Outport
  wires:
  in/1 -> out/1

== system test_mdl_NI/CAN_Signal/GWM/Other_GWMTx/Body_Info_9_FD1/CrnkInhbt_B_Stat ==
  in : Inport
  out : Outport
  wires:
  in/1 -> out/1

== system test_mdl_NI/CAN_Signal/GWM/Other_GWMTx/Body_Info_9_FD1/CrnkInhbt_No_Cnt ==
  in : Inport
  out : Outport
  wires:
  in/1 -> out/1

== system test_mdl_NI/CAN_Signal/GWM/Other_GWMTx/Body_Info_9_FD1/CrnkInhbt_No_Cs ==
  in : Inport
  out : Outport
  wires:
  in/1 -> out/1

== system test_mdl_NI/CAN_Signal/GWM/Other_GWMTx/Body_Info_9_FD1/DrvInCtl_B_Stat ==
  in : Inport
  out : Outport
  wires:
  in/1 -> out/1

== system test_mdl_NI/CAN_Signal/GWM/Other_GWMTx/Body_Info_9_FD1/EngStrtActv_B_Stat ==
  in : Inport
  out : Outport
  wires:
  in/1 -> out/1

== system test_mdl_NI/CAN_Signal/GWM/Other_GWMTx/Body_Info_9_FD1/EngStrt_B_Rq ==
  in : Inport
  out : Outport
  wires:
  in/1 -> out/1

== system test_mdl_NI/CAN_Signal/GWM/Other_GWMTx/Body_Info_9_FD1/IgnPreOffActv_B_Stat ==
  in : Inport
  out : Outport
  wires:
  in/1 -> out/1

== system test_mdl_NI/CAN_Signal/GWM/Other_GWMTx/Body_Info_9_FD1/StrtrMtrCtlDStat_No_Cs ==
  in : Inport
  out : Outport
  wires:
  in/1 -> out/1

== system test_mdl_NI/CAN_Signal/GWM/Other_GWMTx/Body_Info_9_FD1/VehOnSrc_D_Stat ==
  in : Inport
  out : Outport
  wires:
  in/1 -> out/1

== system test_mdl_NI/CAN_Signal/GWM/Other_GWMTx/Climate_Cntrl_Data_2_FD1/ApaSwtch_D_RqDrv ==
  in : Inport
  out : Outport
  wires:
  in/1 -> out/1

== system test_mdl_NI/CAN_Signal/GWM/Other_GWMTx/Climate_Cntrl_Data_2_FD1/ApaSwtch_No_Cnt ==
  in : Inport
  out : Outport
  wires:
  in/1 -> out/1

== system test_mdl_NI/CAN_Signal/GWM/Other_GWMTx/Climate_Cntrl_Data_2_FD1/CabnAmb_Te_Actl ==
  in : Inport
  out : Outport
  wires:
  in/1 -> out/1

== system test_mdl_NI/CAN_Signal/GWM/Other_GWMTx/Climate_Cntrl_Data_2_FD1/CamraDefog_B_Actl ==
  in : Inport
  out : Outport
  wires:
  in/1 -> out/1

== system test_mdl_NI/CAN_Signal/GWM/Other_GWMTx/Climate_Cntrl_Data_2_FD1/ClimtThrmlLoad_No_Actl ==
  in : Inport
  out : Outport
  wires:
  in/1 -> out/1

== system test_mdl_NI/CAN_Signal/GWM/Other_GWMTx/Climate_Cntrl_Data_2_FD1/EcoMde_D_RqDrv ==
  in : Inport
  out : Outport
  wires:
  in/1 -> out/1

== system test_mdl_NI/CAN_Signal/GWM/Other_GWMTx/Climate_Cntrl_Data_2_FD1/HvacAir_Flw_Est ==
  in : Inport
  out : Outport
  wires:
  in/1 -> out/1

== system test_mdl_NI/CAN_Signal/GWM/Other_GWMTx/Climate_Cntrl_Data_2_FD1/HvacBlwrFront_D_Stat ==
  in : Inport
  out : Outport
  wires:
  in/1 -> out/1

== system test_mdl_NI/CAN_Signal/GWM/Other_GWMTx/Climate_Cntrl_Data_2_FD1/HvacBlwrRear_D_Stat ==
  in : Inport
  out : Outport
  wires:
  in/1 -> out/1

== system test_mdl_NI/CAN_Signal/GWM/Other_GWMTx/Climate_Cntrl_Data_2_FD1/HvacRec_Pc_Est ==
  in : Inport
  out : Outport
  wires:
  in/1 -> out/1

== system test_mdl_NI/CAN_Signal/GWM/Other_GWMTx/Climate_Cntrl_Data_2_FD1/HvacRemoteStrt_N_Rq ==
  in : Inport
  out : Outport
  wires:
  in/1 -> out/1

== system test_mdl_NI/CAN_Signal/GWM/Other_GWMTx/Climate_Cntrl_Data_2_FD1/TwHlGrdAsst_B_RqTrn ==
  in : Inport
  out : Outport
  wires:
  in/1 -> out/1

== system test_mdl_NI/CAN_Signal/GWM/Other_GWMTx/Climate_Control_Data_FD1/AutoHoldSwtch_D_Stat ==
  in : Inport
  out : Outport
  wires:
  in/1 -> out/1

== system test_mdl_NI/CAN_Signal/GWM/Other_GWMTx/Climate_Control_Data_FD1/CamraFrntBttn_D_Stat ==
  in : Inport
  out : Outport
  wires:
  in/1 -> out/1

== system test_mdl_NI/CAN_Signal/GWM/Other_GWMTx/Climate_Control_Data_FD1/CamraRearBttn_D_Stat ==
  in : Inport
  out : Outport
  wires:
  in/1 -> out/1

== system test_mdl_NI/CAN_Signal/GWM/Other_GWMTx/Climate_Control_Data_FD1/DrvSlipCtlMde_B_Rq ==
  in : Inport
  out : Outport
  wires:
  in/1 -> out/1

== system test_mdl_NI/CAN_Signal/GWM/Other_GWMTx/Climate_Control_Data_FD1/EcoInhbt_B_RqHvac ==
  in : Inport
  out : Outport
  wires:
  in/1 -> out/1

== system test_mdl_NI/CAN_Signal/GWM/Other_GWMTx/Climate_Control_Data_FD1/GlvBoxRleas_No_Actl ==
  in : Inport
  out : Outport
  wires:
  in/1 -> out/1

== system test_mdl_NI/CAN_Signal/GWM/Other_GWMTx/Climate_Control_Data_FD1/LpdbAuxBlwr_B_Rq ==
  in : Inport
  out : Outport
  wires:
  in/1 -> out/1

== system test_mdl_NI/CAN_Signal/GWM/Other_GWMTx/Climate_Control_Data_FD1/LpdbDfrstFlOn_B_Rq ==
  in : Inport
  out : Outport
  wires:
  in/1 -> out/1

== system test_mdl_NI/CAN_Signal/GWM/Other_GWMTx/Climate_Control_Data_FD1/LpdbDfrstFrOn_B_Rq ==
  in : Inport
  out : Outport
  wires:
  in/1 -> out/1

== system test_mdl_NI/CAN_Signal/GWM/Other_GWMTx/Climate_Control_Data_FD1/LpdbDfrstRearOn_B_Rq ==
  in : Inport
  out : Outport
  wires:
  in/1 -> out/1

== system test_mdl_NI/CAN_Signal/GWM/Other_GWMTx/Climate_Control_Data_FD1/LpdbHeatWiprPrk_B_Rq ==
  in : Inport
  out : Outport
  wires:
  in/1 -> out/1

== system test_mdl_NI/CAN_Signal/GWM/Other_GWMTx/Climate_Control_Data_FD1/LpdbPtc1_B_Rq ==
  in : Inport
  out : Outport
  wires:
  in/1 -> out/1

== system test_mdl_NI/CAN_Signal/GWM/Other_GWMTx/Climate_Control_Data_FD1/LpdbPtc2_B_Rq ==
  in : Inport
  out : Outport
  wires:
  in/1 -> out/1

== system test_mdl_NI/CAN_Signal/GWM/Other_GWMTx/Climate_Control_Data_FD1/LpdbPtc3_B_Rq ==
  in : Inport
  out : Outport
  wires:
  in/1 -> out/1

== system test_mdl_NI/CAN_Signal/GWM/Other_GWMTx/Climate_Control_Data_FD1/MirrorHeatOn_B_Rq ==
  in : Inport
  out : Outport
  wires:
  in/1 -> out/1

== system test_mdl_NI/CAN_Signal/GWM/Other_GWMTx/Climate_Control_Data_FD1/Outside_Air_Temp_Stat ==
  in : Inport
  out : Outport
  wires:
  in/1 -> out/1

== system test_mdl_NI/CAN_Signal/GWM/Other_GWMTx/Climate_Control_Data_FD1/PrkAidSwtch_D_RqDrv ==
  in : Inport
  out : Outport
  wires:
  in/1 -> out/1

== system test_mdl_NI/CAN_Signal/GWM/Other_GWMTx/Climate_Control_Data_FD1/PrkAidSwtch_No_Cnt ==
  in : Inport
  out : Outport
  wires:
  in/1 -> out/1

== system test_mdl_NI/CAN_Signal/GWM/Other_GWMTx/Climate_Control_Data_FD1/Remote_Start_QuietMode ==
  in : Inport
  out : Outport
  wires:
  in/1 -> out/1

== system test_mdl_NI/CAN_Signal/GWM/Other_GWMTx/Climate_Control_Data_FD1/SteWhlHeat_D_Rq ==
  in : Inport
  out : Outport
  wires:
  in/1 -> out/1

== system test_mdl_NI/CAN_Signal/GWM/Other_GWMTx/Climate_Control_Data_FD1/TrailCtlSwtch_B_Stat ==
  in : Inport
  out : Outport
  wires:
  in/1 -> out/1

== system test_mdl_NI/CAN_Signal/GWM/Other_GWMTx/Cluster_Info1_FD1/AccDeny_B_RqIpc ==
  in : Inport
  out : Outport
  wires:
  in/1 -> out/1

== system test_mdl_NI/CAN_Signal/GWM/Other_GWMTx/Cluster_Info1_FD1/AccEnbl_B_RqDrv ==
  in : Inport
  out : Outport
  wires:
  in/1 -> out/1

== system test_mdl_NI/CAN_Signal/GWM/Other_GWMTx/Cluster_Info1_FD1/BulbChkActv_B_Stat ==
  in : Inport
  out : Outport
  wires:
  in/1 -> out/1

== system test_mdl_NI/CAN_Signal/GWM/Other_GWMTx/Cluster_Info1_FD1/DrvPerfMde_D_Rq ==
  in : Inport
  out : Outport
  wires:
  in/1 -> out/1

== system test_mdl_NI/CAN_Signal/GWM/Other_GWMTx/Cluster_Info1_FD1/DrvSlipCtlMde_B_Rq2 ==
  in : Inport
  out : Outport
  wires:
  in/1 -> out/1

== system test_mdl_NI/CAN_Signal/GWM/Other_GWMTx/Cluster_Info1_FD1/DrvSlipCtlMde_D_Rq ==
  in : Inport
  out : Outport
  wires:
  in/1 -> out/1

== system test_mdl_NI/CAN_Signal/GWM/Other_GWMTx/Cluster_Info1_FD1/EmgcyCallAsstMykey_Rq ==
  in : Inport
  out : Outport
  wires:
  in/1 -> out/1

== system test_mdl_NI/CAN_Signal/GWM/Other_GWMTx/Cluster_Info1_FD1/EngIdlShutDown_B_RqDrv ==
  in : Inport
  out : Outport
  wires:
  in/1 -> out/1

== system test_mdl_NI/CAN_Signal/GWM/Other_GWMTx/Cluster_Info1_FD1/EngOilLife_B_RqReset ==
  in : Inport
  out : Outport
  wires:
  in/1 -> out/1

== system test_mdl_NI/CAN_Signal/GWM/Other_GWMTx/Cluster_Info1_FD1/Fda_B_Stat ==
  in : Inport
  out : Outport
  wires:
  in/1 -> out/1

== system test_mdl_NI/CAN_Signal/GWM/Other_GWMTx/Cluster_Info1_FD1/FrostWarn_D_Stat ==
  in : Inport
  out : Outport
  wires:
  in/1 -> out/1

== system test_mdl_NI/CAN_Signal/GWM/Other_GWMTx/Cluster_Info1_FD1/HsaMde_D_Rq ==
  in : Inport
  out : Outport
  wires:
  in/1 -> out/1

== system test_mdl_NI/CAN_Signal/GWM/Other_GWMTx/Cluster_Info1_FD1/KeyTypeChngMykey_D_Rq ==
  in : Inport
  out : Outport
  wires:
  in/1 -> out/1

== system test_mdl_NI/CAN_Signal/GWM/Other_GWMTx/Cluster_Info1_FD1/LscmbbStat_B_Actl ==
  in : Inport
  out : Outport
  wires:
  in/1 -> out/1

== system test_mdl_NI/CAN_Signal/GWM/Other_GWMTx/Cluster_Info1_FD1/ManRgen_D_Rq ==
  in : Inport
  out : Outport
  wires:
  in/1 -> out/1

== system test_mdl_NI/CAN_Signal/GWM/Other_GWMTx/Cluster_Info1_FD1/MetricActvTe_B_Actl ==
  in : Inport
  out : Outport
  wires:
  in/1 -> out/1

== system test_mdl_NI/CAN_Signal/GWM/Other_GWMTx/Cluster_Info1_FD1/MetricActv_B_Actl ==
  in : Inport
  out : Outport
  wires:
  in/1 -> out/1

== system test_mdl_NI/CAN_Signal/GWM/Other_GWMTx/Cluster_Info1_FD1/NtrlTowMdeEnbl_B_RqDrv ==
  in : Inport
  out : Outport
  wires:
  in/1 -> out/1

== system test_mdl_NI/CAN_Signal/GWM/Other_GWMTx/Cluster_Info1_FD1/OdometerMasterValue ==
  in : Inport
  out : Outport
  wires:
  in/1 -> out/1

== system test_mdl_NI/CAN_Signal/GWM/Other_GWMTx/Cluster_Info1_FD1/ParkDetect_Stat ==
  in : Inport
  out : Outport
  wires:
  in/1 -> out/1

== system test_mdl_NI/CAN_Signal/GWM/Other_GWMTx/Cluster_Info1_FD1/Power_Liftgate_Mode_Cmd ==
  in : Inport
  out : Outport
  wires:
  in/1 -> out/1

== system test_mdl_NI/CAN_Signal/GWM/Other_GWMTx/Cluster_Info1_FD1/PrkLckCtlEnbl_D_RqIpc ==
  in : Inport
  out : Outport
  wires:
  in/1 -> out/1

== system test_mdl_NI/CAN_Signal/GWM/Other_GWMTx/Cluster_Info1_FD1/PtDrvMde_D_Rq ==
  in : Inport
  out : Outport
  wires:
  in/1 -> out/1

== system test_mdl_NI/CAN_Signal/GWM/Other_GWMTx/Cluster_Info1_FD1/ReducedGuard_D_Rq ==
  in : Inport
  out : Outport
  wires:
  in/1 -> out/1

== system test_mdl_NI/CAN_Signal/GWM/Other_GWMTx/Cluster_Info1_FD1/StopStrtDrvMde_D_RqMnu ==
  in : Inport
  out : Outport
  wires:
  in/1 -> out/1

== system test_mdl_NI/CAN_Signal/GWM/Other_GWMTx/Cluster_Info1_FD1/TRAILER_BRAKE_CONFIG ==
  in : Inport
  out : Outport
  wires:
  in/1 -> out/1

== system test_mdl_NI/CAN_Signal/GWM/Other_GWMTx/Cluster_Info1_FD1/TRLR_SWAY_CONFIG_CMD ==
  in : Inport
  out : Outport
  wires:
  in/1 -> out/1

== system test_mdl_NI/CAN_Signal/GWM/Other_GWMTx/Cluster_Info1_FD1/TrlrBrkMde_D_Rq ==
  in : Inport
  out : Outport
  wires:
  in/1 -> out/1

== system test_mdl_NI/CAN_Signal/GWM/Other_GWMTx/Cluster_Info1_FD1/ePRNDL_MODE ==
  in : Inport
  out : Outport
  wires:
  in/1 -> out/1

== system test_mdl_NI/CAN_Signal/GWM/Other_GWMTx/Cluster_Info_3_FD1/AutoRgen_D_Rq ==
  in : Inport
  out : Outport
  wires:
  in/1 -> out/1

== system test_mdl_NI/CAN_Signal/GWM/Other_GWMTx/Cluster_Info_3_FD1/DISPLAY_SPEED_OFFSET ==
  in : Inport
  out : Outport
  wires:
  in/1 -> out/1

== system test_mdl_NI/CAN_Signal/GWM/Other_GWMTx/Cluster_Info_3_FD1/DISPLAY_SPEED_SCALING ==
  in : Inport
  out : Outport
  wires:
  in/1 -> out/1

== system test_mdl_NI/CAN_Signal/GWM/Other_GWMTx/Cluster_Info_3_FD1/DrvSlipCtlMde_B_RqMyKey ==
  in : Inport
  out : Outport
  wires:
  in/1 -> out/1

== system test_mdl_NI/CAN_Signal/GWM/Other_GWMTx/Cluster_Info_3_FD1/FUEL_SENSOR_NUM ==
  in : Inport
  out : Outport
  wires:
  in/1 -> out/1

== system test_mdl_NI/CAN_Signal/GWM/Other_GWMTx/Cluster_Info_3_FD1/FuelLvlActvSide_No_Raw ==
  in : Inport
  out : Outport
  wires:
  in/1 -> out/1

== system test_mdl_NI/CAN_Signal/GWM/Other_GWMTx/Cluster_Info_3_FD1/FuelLvlPssvSide_No_Raw ==
  in : Inport
  out : Outport
  wires:
  in/1 -> out/1

== system test_mdl_NI/CAN_Signal/GWM/Other_GWMTx/Cluster_Info_3_FD1/FuelLvlWarn_D_Actl ==
  in : Inport
  out : Outport
  wires:
  in/1 -> out/1

== system test_mdl_NI/CAN_Signal/GWM/Other_GWMTx/Cluster_Info_3_FD1/FuelLvl_Pc_Dsply ==
  in : Inport
  out : Outport
  wires:
  in/1 -> out/1

== system test_mdl_NI/CAN_Signal/GWM/Other_GWMTx/Cluster_Info_3_FD1/FuelSecndActv_B_Actl ==
  in : Inport
  out : Outport
  wires:
  in/1 -> out/1

== system test_mdl_NI/CAN_Signal/GWM/Other_GWMTx/Cluster_Info_3_FD1/OdoTripRx_B_Actl ==
  in : Inport
  out : Outport
  wires:
  in/1 -> out/1

== system test_mdl_NI/CAN_Signal/GWM/Other_GWMTx/Cluster_Info_3_FD1/Veh_V_CompLimMx ==
  in : Inport
  out : Outport
  wires:
  in/1 -> out/1

== system test_mdl_NI/CAN_Signal/GWM/Other_GWMTx/Cluster_Info_3_FD1/W2S_LAMP_OK ==
  in : Inport
  out : Outport
  wires:
  in/1 -> out/1

== system test_mdl_NI/CAN_Signal/GWM/Other_GWMTx/Cluster_Lighting_Rq_FD1/IsaOffst_D_Rq ==
  in : Inport
  out : Outport
  wires:
  in/1 -> out/1

== system test_mdl_NI/CAN_Signal/GWM/Other_GWMTx/Cluster_Lighting_Rq_FD1/SlMde_D_Rq ==
  in : Inport
  out : Outport
  wires:
  in/1 -> out/1

== system test_mdl_NI/CAN_Signal/GWM/Other_GWMTx/Compressor_Req_FD1/ClimtCoolRear_B_Rq ==
  in : Inport
  out : Outport
  wires:
  in/1 -> out/1

== system test_mdl_NI/CAN_Signal/GWM/Other_GWMTx/Compressor_Req_FD1/ClimtCool_D_Rq ==
  in : Inport
  out : Outport
  wires:
  in/1 -> out/1

== system test_mdl_NI/CAN_Signal/GWM/Other_GWMTx/Compressor_Req_FD1/ClimtDeltaLoad_Pw_Actl ==
  in : Inport
  out : Outport
  wires:
  in/1 -> out/1

== system test_mdl_NI/CAN_Signal/GWM/Other_GWMTx/Compressor_Req_FD1/ClimtHeatRear_D_Rq ==
  in : Inport
  out : Outport
  wires:
  in/1 -> out/1

== system test_mdl_NI/CAN_Signal/GWM/Other_GWMTx/Compressor_Req_FD1/ClimtHeat_D_Rq ==
  in : Inport
  out : Outport
  wires:
  in/1 -> out/1

== system test_mdl_NI/CAN_Signal/GWM/Other_GWMTx/Compressor_Req_FD1/ClimtPw_B_Rq ==
  in : Inport
  out : Outport
  wires:
  in/1 -> out/1

== system test_mdl_NI/CAN_Signal/GWM/Other_GWMTx/Compressor_Req_FD1/HtrCorePump_B_Rq ==
  in : Inport
  out : Outport
  wires:
  in/1 -> out/1

== system test_mdl_NI/CAN_Signal/GWM/Other_GWMTx/Compressor_Req_FD1/HvacAirCond_B_Rq ==
  in : Inport
  out : Outport
  wires:
  in/1 -> out/1

== system test_mdl_NI/CAN_Signal/GWM/Other_GWMTx/Compressor_Req_FD1/HvacEvap_Te_Actl ==
  in : Inport
  out : Outport
  wires:
  in/1 -> out/1

== system test_mdl_NI/CAN_Signal/GWM/Other_GWMTx/Compressor_Req_FD1/HvacEvap_Te_Offst ==
  in : Inport
  out : Outport
  wires:
  in/1 -> out/1

== system test_mdl_NI/CAN_Signal/GWM/Other_GWMTx/Compressor_Req_FD1/HvacEvap_Te_Rq ==
  in : Inport
  out : Outport
  wires:
  in/1 -> out/1

== system test_mdl_NI/CAN_Signal/GWM/Other_GWMTx/Compressor_Req_FD1/HvacHtrCore_Te_Rq ==
  in : Inport
  out : Outport
  wires:
  in/1 -> out/1

== system test_mdl_NI/CAN_Signal/GWM/Other_GWMTx/Compressor_Req_FD1/SnowPlowMde_B_Enbl ==
  in : Inport
  out : Outport
  wires:
  in/1 -> out/1

== system test_mdl_NI/CAN_Signal/GWM/Other_GWMTx/Compressor_Req_FD1/StopStrtDrvMde_B_RqBtn ==
  in : Inport
  out : Outport
  wires:
  in/1 -> out/1

== system test_mdl_NI/CAN_Signal/GWM/Other_GWMTx/Compressor_Req_FD1/WndwFrontHeat_B_Stat ==
  in : Inport
  out : Outport
  wires:
  in/1 -> out/1

== system test_mdl_NI/CAN_Signal/GWM/Other_GWMTx/CruiseCtrl_Strg_Data_FD1/AccButtnGapDecPress2 ==
  in : Inport
  out : Outport
  wires:
  in/1 -> out/1

== system test_mdl_NI/CAN_Signal/GWM/Other_GWMTx/CruiseCtrl_Strg_Data_FD1/AccButtnGapIncPress2 ==
  in : Inport
  out : Outport
  wires:
  in/1 -> out/1

== system test_mdl_NI/CAN_Signal/GWM/Other_GWMTx/CruiseCtrl_Strg_Data_FD1/AccButtnGpTogglePress2 ==
  in : Inport
  out : Outport
  wires:
  in/1 -> out/1

== system test_mdl_NI/CAN_Signal/GWM/Other_GWMTx/CruiseCtrl_Strg_Data_FD1/ActvFrontSteLck_D_Stat ==
  in : Inport
  out : Outport
  wires:
  in/1 -> out/1

== system test_mdl_NI/CAN_Signal/GWM/Other_GWMTx/CruiseCtrl_Strg_Data_FD1/ActvFrontSteMsgTxt_D_Rq ==
  in : Inport
  out : Outport
  wires:
  in/1 -> out/1

== system test_mdl_NI/CAN_Signal/GWM/Other_GWMTx/CruiseCtrl_Strg_Data_FD1/AslButtnOnOffCnclPres2 ==
  in : Inport
  out : Outport
  wires:
  in/1 -> out/1

== system test_mdl_NI/CAN_Signal/GWM/Other_GWMTx/CruiseCtrl_Strg_Data_FD1/AslButtnOnOffPress2 ==
  in : Inport
  out : Outport
  wires:
  in/1 -> out/1

== system test_mdl_NI/CAN_Signal/GWM/Other_GWMTx/CruiseCtrl_Strg_Data_FD1/CcAslButtnCnclPress2 ==
  in : Inport
  out : Outport
  wires:
  in/1 -> out/1

== system test_mdl_NI/CAN_Signal/GWM/Other_GWMTx/CruiseCtrl_Strg_Data_FD1/CcAslButtnCnclResPres2 ==
  in : Inport
  out : Outport
  wires:
  in/1 -> out/1

== system test_mdl_NI/CAN_Signal/GWM/Other_GWMTx/CruiseCtrl_Strg_Data_FD1/CcAslButtnDeny_B_Actl2 ==
  in : Inport
  out : Outport
  wires:
  in/1 -> out/1

== system test_mdl_NI/CAN_Signal/GWM/Other_GWMTx/CruiseCtrl_Strg_Data_FD1/CcAslButtnIndxDecPres2 ==
  in : Inport
  out : Outport
  wires:
  in/1 -> out/1

== system test_mdl_NI/CAN_Signal/GWM/Other_GWMTx/CruiseCtrl_Strg_Data_FD1/CcAslButtnIndxIncPres2 ==
  in : Inport
  out : Outport
  wires:
  in/1 -> out/1

== system test_mdl_NI/CAN_Signal/GWM/Other_GWMTx/CruiseCtrl_Strg_Data_FD1/CcAslButtnOffCnclPres2 ==
  in : Inport
  out : Outport
  wires:
  in/1 -> out/1

== system test_mdl_NI/CAN_Signal/GWM/Other_GWMTx/CruiseCtrl_Strg_Data_FD1/CcAslButtnOnOffCncl2 ==
  in : Inport
  out : Outport
  wires:
  in/1 -> out/1

== system test_mdl_NI/CAN_Signal/GWM/Other_GWMTx/CruiseCtrl_Strg_Data_FD1/CcAslButtnOnPress2 ==
  in : Inport
  out : Outport
  wires:
  in/1 -> out/1

== system test_mdl_NI/CAN_Signal/GWM/Other_GWMTx/CruiseCtrl_Strg_Data_FD1/CcAslButtnResDecPress2 ==
  in : Inport
  out : Outport
  wires:
  in/1 -> out/1

== system test_mdl_NI/CAN_Signal/GWM/Other_GWMTx/CruiseCtrl_Strg_Data_FD1/CcAslButtnResIncPress2 ==
  in : Inport
  out : Outport
  wires:
  in/1 -> out/1
